simulink model "Electronic_Throttle_Control"  (R2024a)
settings: Solver=VariableStepDiscrete  StartTime=0.0  StopTime=10.0  RelTol=1e-3
settings Model: Creator=DELL  LastModifiedBy=DELL
settings DataIOCC: LoadExternalInput=on

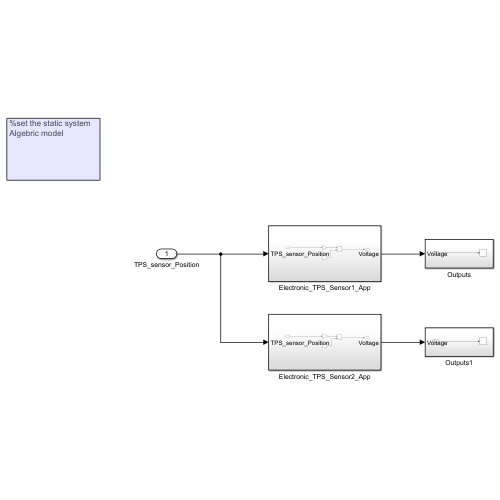
[thumbnail: Simulink's stored preview of the top-level diagram]
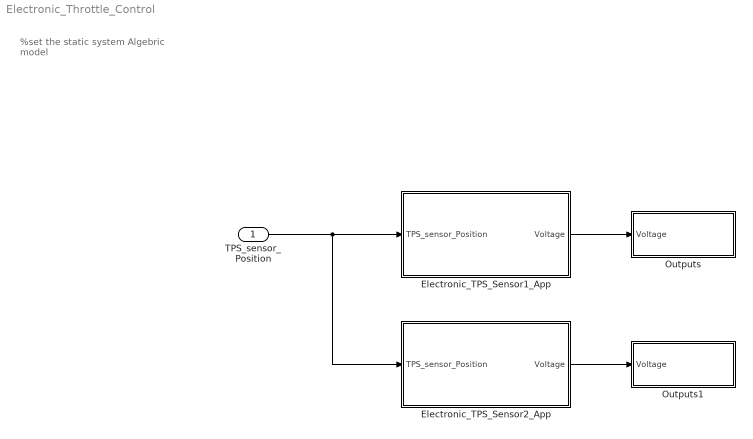
== system Electronic_Throttle_Control ==
  note: %set the static system
      | Algebric model
  TPS_sensor_Position : Inport
  Electronic_TPS_Sensor1_App : Subsystem
  Electronic_TPS_Sensor2_App : Subsystem
  Outputs : Subsystem
  Outputs1 : Subsystem
  wires:
  Electronic_TPS_Sensor1_App/1(Voltage) -> Outputs/1(Voltage)
  TPS_sensor_Position/1 -> Electronic_TPS_Sensor2_App/1(TPS_sensor_Position), Electronic_TPS_Sensor1_App/1(TPS_sensor_Position)
  Electronic_TPS_Sensor2_App/1(Voltage) -> Outputs1/1(Voltage)

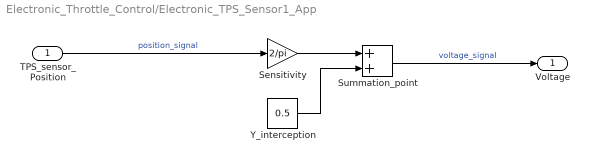
== system Electronic_Throttle_Control/Electronic_TPS_Sensor1_App ==
  TPS_sensor_Position : Inport
  Sensitivity : Gain  Gain=2/pi
  Summation_point : Sum
  Y_interception : Constant  Value=0.5
  Voltage : Outport
  wires:
  Sensitivity/1 -> Summation_point/1
  Y_interception/1 -> Summation_point/2
  TPS_sensor_Position/1 -> Sensitivity/1  "position_signal"
  Summation_point/1 -> Voltage/1  "voltage_signal"

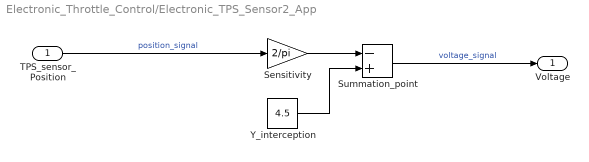
== system Electronic_Throttle_Control/Electronic_TPS_Sensor2_App ==
  TPS_sensor_Position : Inport
  Sensitivity : Gain  Gain=2/pi
  Summation_point : Sum  Inputs=-+
  Y_interception : Constant  Value=4.5
  Voltage : Outport
  wires:
  Summation_point/1 -> Voltage/1  "voltage_signal"
  TPS_sensor_Position/1 -> Sensitivity/1  "position_signal"
  Y_interception/1 -> Summation_point/2
  Sensitivity/1 -> Summation_point/1

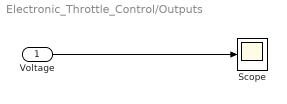
== system Electronic_Throttle_Control/Outputs ==
  Voltage : Inport
  Scope : Scope
  wires:
  Voltage/1 -> Scope/1

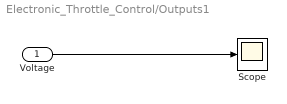
== system Electronic_Throttle_Control/Outputs1 ==
  Voltage : Inport
  Scope : Scope
  wires:
  Voltage/1 -> Scope/1
